simulink model "AutonomousTemplate_2020a"  (R2020a)
settings: Solver=ode23t  StartTime=0.0  StopTime=180.1  FixedStep=0.05  RelTol=1e-3  EnableMultiTasking=on
model workspace (MAT data in the model file):
  mapForSim : object (value not decoded)
  occGrid : robotics.BinaryOccupancyGrid (value not decoded)
undefined symbols (not defined in the file): cellLevel, cellPose, cellTypeArray, FloorSurface, isoPoses, platformPoses, PlowSurface, Ref, RobotSurface, WallSurface, X, Y, Z
libraries: sm_lib x286, nesl_utility x157, simulink x72, vexcommonlib x1
(part 15 of 15)

== stateflow chart AutonomousTemplate_2020a/Flow for robot movement ==
  note: At this point the Robot has done the entire left side for the field (looking out for where the robot start at) and needs to get to the left side. This is what this does
  note: This move the robot to the first box of cells and quickly moves into the movement program.
  state dispose3
    lach=0;
  state START
    Rmotor=0;
    Lmotor=0;
    scolev=1;
    i=0;
    tim=0;
    kim=0;
    c=0;
    cellin=0;
    lach=0;
    vac = 0;
    VCheck = 0;
  state Forward
    Rmotor=100;
    Lmotor=100;
  state Stop
    Rmotor = 0;
    Lmotor=0;
    scolev=0;
  state dispose1
    lach=0;
  note: After the robot does the sweep program before this it becomes a little off-center and need to return to the middle and that is done here.
  state dispose
    lach=0;
  state check7
    Rmotor=-50;
    Lmotor=50;
  state quit3
    Rmotor=0;
    Lmotor=0;
  state check3
    Rmotor=-50;
    Lmotor=50;
  state quit1
    Rmotor=0;
    Lmotor=0;
  note: After the robot does the sweep program before this it becomes a little off-center and need to return to the middle and that is done here.
  state Stop9
    Rmotor = 0;
    Lmotor=0;
  note: Second box isolating
  state Turn190
    Rmotor=27;
    Lmotor=-27;
  state Turn189
    Rmotor=29;
    Lmotor=-29;
  state Stop74
    Rmotor=0;
    Lmotor=0;
    lach=0;
  state Turn188
    Rmotor=29;
    Lmotor=-29;
  state correct
    Lmotor=25;
    Rmotor=0;
  state check1
    Rmotor=-50;
    Lmotor=50;
  state quit
    Rmotor=0;
    Lmotor=0;
  state dispose2
    lach=0;
  note: After the robot does the sweep program before this it becomes a little off-center and need to return to the middle and that is done here.
  state wat3
    Rmotor=0;
    Lmotor=0
  state Turn185
    Rmotor=27;
    Lmotor=-27;
  state Turn184
    Rmotor=29;
    Lmotor=-29;
  state Stop70
    Rmotor=0;
    Lmotor=0;
    lach=0;
  state Turn186
    Rmotor=29;
    Lmotor=-29;
  state Forward1
    Rmotor=50
    Lmotor=50;
    scolev=1;
  state Stop4
    Rmotor = 0;
    Lmotor=0;
  state Backwards
    Rmotor=-30;
    Lmotor=-30;
    scolev=0;
  state Stop6
    Rmotor = 0;
    Lmotor=0;
  state wat1
    Rmotor=0;
    Lmotor=0
  state Stop73
    Rmotor=50;
    Lmotor=50;
  state Turn191
    Rmotor=29;
    Lmotor=-29;
  state wat
    Rmotor=0;
    Lmotor=0
  state check5
    Rmotor=-50;
    Lmotor=50;
  state quit2
    Rmotor=0;
    Lmotor=0;
  state correct5
    Lmotor=25;
    Rmotor=0;
  state return1
    Lmotor=20;
    Rmotor=0;
  state Stop14
    Rmotor = 0;
    Lmotor=0;
  state check6
    Rmotor=50;
    Lmotor=-50;
  state Stop69
    Rmotor=0;
    Lmotor=0;
  state Turn187
    Rmotor=29;
    Lmotor=-29;
  state check2
    Rmotor=50;
    Lmotor=-50;
  state correct2
    Lmotor=25;
    Rmotor=0;
  state return
    Lmotor=20;
    Rmotor=0;
  state Stop12
    Rmotor = 0;
    Lmotor=0;
  note: It may seem that this 1 sec is not neceisary, but If I were to instantly transfer into the next state it would mess up my perfect 90-degree angle.
  note: after(1.4,sec)
  state check
    Rmotor=50;
    Lmotor=-50;
  state wat2
    Rmotor=0;
    Lmotor=0
  state drop
    Rmotor=50
    Lmotor=50;
    lach=0;
  state Turn90
    Rmotor=28.5;
    Lmotor=-28.5;
  state Stop5
    Rmotor = 0;
    Lmotor=0;
  state Vaccine
    vac = 1;
    Rmotor = 50;
    Lmotor = 50;
  state correct1
    Lmotor=0;
    Rmotor=25;
  state Backwards1
    Rmotor=-30;
    Lmotor=-30;
    scolev=0;
  state Vaccine3
    vac = 1;
    Rmotor = 50;
    Lmotor = 50;
  state Stop72
    Rmotor=50;
    Lmotor=50;
  state Vaccine1
    vac = 1;
    Rmotor = 50;
    Lmotor = 50;
  state check4
    Rmotor=50;
    Lmotor=-50;
  state Stop71
    Rmotor=0;
    Lmotor=0;
  state correct4
    Lmotor=0;
    Rmotor=25;
  state Backwards3
    Rmotor=-30;
    Lmotor=-30;
    scolev=0;
  state Vaccinate3
    Rmotor = -50;
    Lmotor = -50;
  state Vaccinate
    Rmotor = -50;
    Lmotor = -50;
  state Vaccinate1
    Rmotor = -50;
    Lmotor = -50;
  state correct3
    Lmotor=0;
    Rmotor=25;
  state Backwards2
    Rmotor=-30;
    Lmotor=-30;
    scolev=0;
  state Vaccine2
    vac = 1;
    Rmotor = 50;
    Lmotor = 50;
  note: This marks the START of the sweep program . The times are almost to the exact. make sure when using this you have the robot start at the correct place. otherwise the sweep will not work (by not covoring all possible spaces the may contain cells)
  note: This marks the START of the sweep program . The times are almost to the exact. make sure when using this you have the robot start at the correct place. otherwise the sweep will not work (by not covoring all possible spaces the may contain cells)
  note: This marks the START of the sweep program . The times are almost to the exact. make sure when using this you have the robot start at the correct place. otherwise the sweep will not work (by not covoring all possible spaces the may contain cells)
  note: This marks the START of the sweep program . The times are almost to the exact. make sure when using this you have the robot start at the correct place. otherwise the sweep will not work (by not covoring all possible spaces the may contain cells)
  note: when I refer to the sweep the dircetion movement refered to by L or R does NOT reflect the direction in which the robot rotates one motor?
  state Vaccinate2
    Rmotor = -50;
    Lmotor = -50;
  note: This marks the END of the sweep program ; when reused change the varibles so that it does not conflict.
  state Stop3
    Rmotor = 0;
    Lmotor=0;
    c=0;
    cellin=0;
    VCheck = 0;
  note: This marks the END of the sweep program ; when reused change the varibles so that it does not conflict.
  state Stop56
    Rmotor = 0;
    Lmotor=0;
    c=0;
    cellin=0;
  state Stop60
    Rmotor = 0;
    Lmotor=0;
    c=0;
    cellin=0;
  note: Troble Shoot
  note: This marks the END of the sweep program ; when reused change the varibles so that it does not conflict.
  state latch105
    i=1;
    lach=1;
    kim=time;
    cellin=1;
  state latch112
    i=1;
    lach=1;
    kim=time;
    cellin=1;
  state latch119
    i=1;
    lach=1;
    kim=time;
    cellin=1;
  state SweepR
    Rmotor=25;
    Lmotor=0;
  state time
    tim=time;
    c = c + 1;
    i=0;
  state SweepR84
    Rmotor=25;
    Lmotor=0;
  state time105
    tim=time;
    c = c + 1;
    i=0;
  state SweepR88
    Rmotor=25;
    Lmotor=0;
  state time112
    tim=time;
    c = c + 1;
    i=0;
  state SweepR92
    Rmotor=25;
    Lmotor=0;
  state time119
    tim=time;
    c = c + 1;
    i=0;
  state latch3
    i=1;
    lach=1;
    kim=time;
    cellin=1;
  state Stop58
    Rmotor = 0;
    Lmotor=0;
    c=0;
    cellin=0;
  state Reset
    Rmotor=50;
    Lmotor=50
    i=0;
  note: This marks the END of the sweep program ; when reused change the varibles so that it does not conflict.
  note: this is speific to this flow only and cannot be used on other sweeps
  state Stop57
    Rmotor = 0;
    Lmotor=0;
  state SweepL
    Rmotor=-22.5;
    Lmotor=25;
  state time1
    tim=time;
    c =c+1;
    i=0;
  state SweepL65
    Rmotor=-22.5;
    Lmotor=25;
  state time111
    tim=time;
    c =c+1;
    i=0;
  state SweepL68
    Rmotor=-22.5;
    Lmotor=25;
  state time118
    tim=time;
    c =c+1;
    i=0;
  state SweepL71
    Rmotor=-22.5;
    Lmotor=25;
  state time125
    tim=time;
    c =c+1;
    i=0;
  state latch106
    i=1;
    lach=1;
    kim=time;
    cellin==1;
  state latch113
    i=1;
    lach=1;
    kim=time;
    cellin==1;
  state latch120
    i=1;
    lach=1;
    kim=time;
    cellin==1;
  state latch
    i=1;
    lach=1;
    kim=time;
    cellin==1;
  state Stop1
    Rmotor = 0;
    Lmotor=0;
  state Stop59
    Rmotor = 0;
    Lmotor=0;
  state Stop61
    Rmotor = 0;
    Lmotor=0;
  note: after(.632,sec)
  state SweepR1
    Rmotor=25;
    Lmotor=-10;
  state time2
    tim=time;
    c = c + 1;
    i=0;
  state SweepR87
    Rmotor=25;
    Lmotor=-10;
  state time107
    tim=time;
    c = c + 1;
    i=0;
  state SweepR91
    Rmotor=25;
    Lmotor=-10;
  state time114
    tim=time;
    c = c + 1;
    i=0;
  state SweepR95
    Rmotor=25;
    Lmotor=-10;
  state time121
    tim=time;
    c = c + 1;
    i=0;
  state latch110
    i=1;
    lach=1;
    kim=time;
    cellin=1;
  state latch117
    i=1;
    lach=1;
    kim=time;
    cellin=1;
  state latch124
    i=1;
    lach=1;
    kim=time;
    cellin=1;
  state latch1
    i=1;
    lach=1;
    kim=time;
    cellin=1;
  state latch107
    i=1;
    lach=1;
    kim=time;
    cellin=1;
  state latch114
    i=1;
    lach=1;
    kim=time;
    cellin=1;
  state latch121
    i=1;
    lach=1;
    kim=time;
    cellin=1;
  state latch6
    i=1;
    lach=1;
    kim=time;
    cellin=1;
  state time4
    tim=time;
    c = c + 1;
    i=0;
  state time6
    tim=time;
    c = c + 1;
    i=0;
  state SweepR3
    Rmotor=25;
    Lmotor=-22.5;
  state time108
    tim=time;
    c = c + 1;
    i=0;
  state time109
    tim=time;
    c = c + 1;
    i=0;
  state SweepR86
    Rmotor=25;
    Lmotor=-22.5;
  state time115
    tim=time;
    c = c + 1;
    i=0;
  state time116
    tim=time;
    c = c + 1;
    i=0;
  state SweepR90
    Rmotor=25;
    Lmotor=-22.5;
  state time122
    tim=time;
    c = c + 1;
    i=0;
  state time123
    tim=time;
    c = c + 1;
    i=0;
  state SweepR94
    Rmotor=25;
    Lmotor=-22.5;
  state latch5
    i=1;
    lach=1;
    kim=time;
    cellin=1;
  state latch108
    i=1;
    lach=1;
    kim=time;
    cellin=1;
  state latch115
    i=1;
    lach=1;
    kim=time;
    cellin=1;
  state latch122
    i=1;
    lach=1;
    kim=time;
    cellin=1;
  state SweepL1
    Rmotor=-22.5;
    Lmotor=25;
  state SweepR2
    Rmotor=25;
    Lmotor=-10;
  state SweepL2
    Rmotor=-22.5;
    Lmotor=25;
  state latch109
    i=1;
    lach=1;
    kim=time;
    cellin=1;
  state SweepL63
    Rmotor=-22.5;
    Lmotor=25;
  state SweepR85
    Rmotor=25;
    Lmotor=-10;
  state SweepL64
    Rmotor=-22.5;
    Lmotor=25;
  state latch116
    i=1;
    lach=1;
    kim=time;
    cellin=1;
  state SweepL66
    Rmotor=-22.5;
    Lmotor=25;
  state SweepR89
    Rmotor=25;
    Lmotor=-10;
  state SweepL67
    Rmotor=-22.5;
    Lmotor=25;
  state latch123
    i=1;
    lach=1;
    kim=time;
    cellin=1;
  state SweepL69
    Rmotor=-22.5;
    Lmotor=25;
  state SweepR93
    Rmotor=25;
    Lmotor=-10;
  state SweepL70
    Rmotor=-22.5;
    Lmotor=25;
  state latch2
    i=1;
    lach=1;
    kim=time;
    cellin=1;
  state time3
    tim=time;
    c = c + 1;
    i=0;
  state time5
    tim=time;
    c = c + 1;
    i=0;
  state time106
    tim=time;
    c = c + 1;
    i=0;
  state latch111
    i=1;
    lach=1;
    kim=time;
    cellin=1;
  state time110
    tim=time;
    c = c + 1;
    i=0;
  state time113
    tim=time;
    c = c + 1;
    i=0;
  state latch118
    i=1;
    lach=1;
    kim=time;
    cellin=1;
  state time117
    tim=time;
    c = c + 1;
    i=0;
  state time120
    tim=time;
    c = c + 1;
    i=0;
  state latch125
    i=1;
    lach=1;
    kim=time;
    cellin=1;
  state time124
    tim=time;
    c = c + 1;
    i=0;
  state latch4
    i=1;
    lach=1;
    kim=time;
    cellin=1;
  state Drop2
    lach = 0;
  state check10
    Rmotor=-50;
    Lmotor=50;
  note: The values are slightly diffrent to account for uncentering during the 180 degree rotation
  note: 3.6 second for next grid line on the specific transition
  state check12
    Rmotor=-50;
    Lmotor=50;
  state check8
    Rmotor=-50;
    Lmotor=50;
  state Rotate2
    Rmotor = 50;
    Lmotor = -50;
  state dispose5
    lach=0;
  state dispose6
    lach=0;
  state Backwards5
    Rmotor=-30;
    Lmotor=-30;
    scolev=0;
  state correct9
    Lmotor=0;
    Rmotor=25;
  state wat5
    Rmotor=0;
    Lmotor=0
  state Forward5
    Rmotor = 50;
    Lmotor = 50;
  state Drop
    lach = 0;
  state Stop17
    Rmotor=0;
    Lmotor=0;
  state Forward2
    Rmotor=50;
    Lmotor=50.7;
  state Turn181
    Rmotor=27;
    Lmotor=-27;
  note: At this point the Robot has done the entire left side for the field (looking out for where the robot start at) and needs to get to the left side. This is what this does
  state Stop24
    Rmotor = 0;
    Lmotor=0;
  state Turn183
    Rmotor=27;
    Lmotor=-27;
  state dispose4
    lach=0;
  state quit5
    Rmotor=0;
    Lmotor=0;
  state wat6
    Rmotor=0;
    Lmotor=0
  state check11
    Rmotor=50;
    Lmotor=-50;
  state Backwards4
    Rmotor=-30;
    Lmotor=-30;
    scolev=0;
  state correct7
    Lmotor=0;
    Rmotor=25;
  state quit6
    Rmotor=0;
    Lmotor=0;
  state wat4
    Rmotor=0;
    Lmotor=0
  state check13
    Rmotor=50;
    Lmotor=-50;
  state Rotate3
    Rmotor = -50;
    Lmotor = 50;
  state Vaccine5
    vac = 1;
    Rmotor = 50;
    Lmotor = 50;
  state quit4
    Rmotor=0;
    Lmotor=0;
  state check9
    Rmotor=50;
    Lmotor=-50;
  state Vaccine6
    vac = 1;
    Rmotor = 50;
    Lmotor = 50;
  note: Had to re-arrange this program to from right to left. refer to here if you need antoher format like this, otherwise use the others.
  state Drop1
    lach = 0;
  state Rotate
    Rmotor = -50;
    Lmotor = 50;
  state Stop16
    Rmotor=0;
    Lmotor=0;
  state Turn182
    Rmotor=29;
    Lmotor=-29;
  state Backwards7
    Rmotor=-30;
    Lmotor=-30;
    scolev=0;
  state correct11
    Lmotor=0;
    Rmotor=25;
  state Rotate1
    Rmotor = 50;
    Lmotor = -50;
  state Vaccinate5
    Rmotor = -50;
    Lmotor = -50;
  state Vaccine4
    vac = 1;
    Rmotor = 50;
    Lmotor = 50;
  state Stop25
    Rmotor = 0;
    Lmotor=0;
  state Backwards6
    Rmotor=-30;
    Lmotor=-30;
    scolev=0;
  state Stop23
    Rmotor = 0;
    Lmotor=0;
  state Forward4
    Lmotor=50;
    Rmotor=50;
  state Stop22
    Rmotor = 0;
    Lmotor=0;
  state correct8
    Lmotor=25;
    Rmotor=0;
  state Vaccinate6
    Rmotor = -50;
    Lmotor = -50;
  state Stop20
    Rmotor = 0;
    Lmotor=0;
  state correct6
    Lmotor=25;
    Rmotor=0;
  note: This marks the START of the sweep program . The times are almost to the exact. make sure when using this you have the robot start at the correct place. otherwise the sweep will not work (by not covoring all possible spaces the may contain cells)
  state Vaccinate4
    Rmotor = -50;
    Lmotor = -50;
  state DropStart
    Rmotor = 50;
    Lmotor = -50;
  state Stop27
    Rmotor = 0;
    Lmotor=0;
  state correct10
    Lmotor=25;
    Rmotor=0;
  state Stop64
    Rmotor = 0;
    Lmotor=0;
    c=0;
    cellin=0;
  note: This marks the END of the sweep program ; when reused change the varibles so that it does not conflict.
  note: This marks the START of the sweep program . The times are almost to the exact. make sure when using this you have the robot start at the correct place. otherwise the sweep will not work (by not covoring all possible spaces the may contain cells)
  state latch133
    i=1;
    lach=1;
    kim=time;
    cellin=1;
  state SweepR103
    Rmotor=25;
    Lmotor=0;
  state time134
    tim=time;
    c = c + 1;
    i=0;
  state Stop62
    Rmotor = 0;
    Lmotor=0;
    c=0;
    cellin=0;
  note: This marks the END of the sweep program ; when reused change the varibles so that it does not conflict.
  note: This marks the START of the sweep program . The times are almost to the exact. make sure when using this you have the robot start at the correct place. otherwise the sweep will not work (by not covoring all possible spaces the may contain cells)
  state Forward6
    Rmotor = 50;
    Lmotor = 50;
  state latch126
    i=1;
    lach=1;
    kim=time;
    cellin=1;
  state SweepR96
    Rmotor=25;
    Lmotor=0;
  state time126
    tim=time;
    c = c + 1;
    i=0;
  state Stop66
    Rmotor = 0;
    Lmotor=0;
    c=0;
    cellin=0;
  note: This marks the END of the sweep program ; when reused change the varibles so that it does not conflict.
  state latch140
    i=1;
    lach=1;
    kim=time;
    cellin=1;
  state SweepR107
    Rmotor=25;
    Lmotor=0;
  state time141
    tim=time;
    c = c + 1;
    i=0;
  state SweepL75
    Rmotor=-22.5;
    Lmotor=25;
  state time133
    tim=time;
    c =c+1;
    i=0;
  state latch139
    i=1;
    lach=1;
    kim=time;
    cellin==1;
  state Drop3
    Rmotor = 0;
    Lmotor = 0;
    lach = 0;
  state Stop65
    Rmotor = 0;
    Lmotor=0;
  state Turn
    Rmotor = 50;
    Lmotor = -50;
  state SweepL74
    Rmotor=-22.5;
    Lmotor=25;
  state time132
    tim=time;
    c =c+1;
    i=0;
  state latch127
    i=1;
    lach=1;
    kim=time;
    cellin==1;
  state Stop63
    Rmotor = 0;
    Lmotor=0;
  state latch138
    i=1;
    lach=1;
    kim=time;
    cellin=1;
  state SweepR102
    Rmotor=25;
    Lmotor=-10;
  state time137
    tim=time;
    c = c + 1;
    i=0;
  state SweepL78
    Rmotor=-22.5;
    Lmotor=25;
  state time140
    tim=time;
    c =c+1;
    i=0;
  state latch135
    i=1;
    lach=1;
    kim=time;
    cellin=1;
  state latch146
    i=1;
    lach=1;
    kim=time;
    cellin==1;
  state SweepR101
    Rmotor=25;
    Lmotor=-22.5;
  state time138
    tim=time;
    c = c + 1;
    i=0;
  state time139
    tim=time;
    c = c + 1;
    i=0;
  state Stop67
    Rmotor = 0;
    Lmotor=0;
  state latch131
    i=1;
    lach=1;
    kim=time;
    cellin=1;
  state SweepR99
    Rmotor=25;
    Lmotor=-10;
  state time128
    tim=time;
    c = c + 1;
    i=0;
  state latch128
    i=1;
    lach=1;
    kim=time;
    cellin=1;
  state SweepR98
    Rmotor=25;
    Lmotor=-22.5;
  state time129
    tim=time;
    c = c + 1;
    i=0;
  state time130
    tim=time;
    c = c + 1;
    i=0;
  state latch134
    i=1;
    lach=1;
    kim=time;
    cellin=1;
  state latch137
    i=1;
    lach=1;
    kim=time;
    cellin=1;
  state SweepL76
    Rmotor=-22.5;
    Lmotor=25;
  state SweepR100
    Rmotor=25;
    Lmotor=-10;
  state SweepL77
    Rmotor=-22.5;
    Lmotor=25;
  state latch145
    i=1;
    lach=1;
    kim=time;
    cellin=1;
  state SweepR106
    Rmotor=25;
    Lmotor=-10;
  state time144
    tim=time;
    c = c + 1;
    i=0;
  state latch142
    i=1;
    lach=1;
    kim=time;
    cellin=1;
  state SweepR105
    Rmotor=25;
    Lmotor=-22.5;
  state time145
    tim=time;
    c = c + 1;
    i=0;
  state time146
    tim=time;
    c = c + 1;
    i=0;
  state latch130
    i=1;
    lach=1;
    kim=time;
    cellin=1;
  state latch129
    i=1;
    lach=1;
    kim=time;
    cellin=1;
  state SweepL73
    Rmotor=-22.5;
    Lmotor=25;
  state SweepR97
    Rmotor=25;
    Lmotor=-10;
  state SweepL72
    Rmotor=-22.5;
    Lmotor=25;
  state latch141
    i=1;
    lach=1;
    kim=time;
    cellin=1;
  state latch144
    i=1;
    lach=1;
    kim=time;
    cellin=1;
  state time136
    tim=time;
    c = c + 1;
    i=0;
  state latch136
    i=1;
    lach=1;
    kim=time;
    cellin=1;
  state time135
    tim=time;
    c = c + 1;
    i=0;
  state SweepL79
    Rmotor=-22.5;
    Lmotor=25;
  state SweepR104
    Rmotor=25;
    Lmotor=-10;
  state SweepL80
    Rmotor=-22.5;
    Lmotor=25;
  state time131
    tim=time;
    c = c + 1;
    i=0;
  state latch132
    i=1;
    lach=1;
    kim=time;
    cellin=1;
  state time127
    tim=time;
    c = c + 1;
    i=0;
  state time143
    tim=time;
    c = c + 1;
    i=0;
  state latch143
    i=1;
    lach=1;
    kim=time;
    cellin=1;
  state time142
    tim=time;
    c = c + 1;
    i=0;
  (default) -> START
  dispose3 -> check7
  dispose1 -> check3
  START -> Forward
  Forward -> Stop : after(2.68,sec)
  quit3 -> correct5 : after(.2,sec)
  wat3 -> dispose3 [order 1] : after(1,sec)[ctype~=2]
  dispose -> check1
  Stop -> SweepR
  wat1 -> dispose1 [order 1] : after(1,sec)[ctype~=2]
  quit1 -> correct : after(.2,sec)
  check7 -> quit3 : after(1,sec)
  wat -> dispose [order 1] : after(1,sec)[ctype==1 || ctype==0]
  check3 -> quit1 : after(1,sec)
  Stop9 -> Turn185 [order 2] : [lach==1]
  quit -> Forward1 : after(.2,sec)
  wat3 -> check7 [order 2] : after(1,sec)[ctype==2]
  dispose2 -> check5
  Stop9 -> SweepR88 [order 1] : [lach==0]
  Stop12 -> Turn190 [order 2] : [lach == 1]
  Stop74 -> Turn188 : after(.2,sec)
  Turn190 -> Turn189 : after(3,sec)
  check1 -> quit : after(1,sec)
  wat1 -> check3 [order 2] : after(1,sec)[ctype==2]
  Stop56 -> correct [order 1] : [lach==0]
  quit2 -> correct2 : after(.2,sec)
  Backwards1 -> Stop9 : after(0.4,sec)
  Turn189 -> Stop73 : [ang<105]
  Stop73 -> Stop74 : after(1.5,sec)
  Turn188 -> Turn191 : after(3,sec)
  Stop70 -> Turn186 : after(.2,sec)
  Turn185 -> Turn184 : after(3,sec)
  correct -> correct1 : after(1,sec)
  wat -> check1 [order 2] : after(1,sec)[ctype==2]
  wat2 -> dispose2 [order 1] : after(1,sec)[ctype~=2]
  drop -> Stop4 : after(.7,sec)
  Backwards -> Stop6 : after(0.85,sec)
  Stop6 -> SweepR84
  Stop3 -> Forward1 [order 1] : [lach==0]
  check6 -> wat3 : after(1,sec)
  Turn184 -> Stop69 : [ang<105]
  Stop69 -> Stop70 : after(.2,sec)
  Turn186 -> Turn187 : after(3,sec)
  check5 -> quit2 : after(1,sec)
  Forward1 -> drop : after(.7,sec)
  Stop4 -> Turn90
  Stop5 -> Backwards : after(0.3,sec)
  Stop60 -> correct5 [order 1] : [lach == 0]
  return1 -> Stop14 : after(.001,sec)
  check2 -> wat1 : after(1,sec)
  Stop14 -> Turn181
  Turn191 -> Stop72 : [ang>75]
  check -> wat : after(1,sec)
  Stop58 -> correct2 [order 1] : [lach == 0]
  wat2 -> check5 [order 2] : after(1,sec)[ctype==2]
  return -> Stop12 : after(.2,sec)
  correct5 -> correct4 : after(1,sec)
  Backwards3 -> return1 : after(.45,sec)
  Stop12 -> SweepR92 [order 1] : [lach == 0]
  Vaccine3 -> check6 : after(1, sec){vac = 0;}
  Turn187 -> Stop71 : [ang>75]
  Vaccine1 -> check2 : after(1, sec){vac = 0;}
  correct2 -> correct3 : after(1,sec)
  Backwards2 -> return : after(.45,sec)
  Vaccine -> check : after(1, sec){vac = 0;}
  Turn90 -> Stop5 : [ang>75]
  check4 -> wat2 : after(1,sec)
  correct1 -> Backwards1 : after(1,sec)
  Stop72 -> SweepR92 : after(1.5, sec)
  Vaccinate -> Vaccine : after(1, sec)
  Vaccinate3 -> Vaccine3 : after(1, sec)
  Stop71 -> SweepR88
  Vaccinate1 -> Vaccine1 : after(1, sec)
  Vaccine2 -> check4 : after(1, sec){vac = 0;}
  correct4 -> Backwards3 : after(1,sec)
  Stop60 -> Vaccinate3 [order 2] : [lach==1]
  correct3 -> Backwards2 : after(1,sec)
  Stop56 -> Vaccinate1 [order 2] : [lach==1]
  Stop3 -> Vaccinate [order 2] : [lach==1]
  Vaccinate2 -> Vaccine2 : after(1, sec)
  Stop58 -> Vaccinate2 [order 2] : [lach==1]
  SweepR84 -> latch105 [order 2] : [cellin==0 && i==0 && ctype==2]
  SweepR88 -> latch112 [order 2] : [cellin==0 && i==0 && ctype==2]
  SweepR92 -> latch119 [order 2] : [cellin==0 && i==0 && ctype==2]
  Stop61 -> Stop60
  SweepR -> time [order 1] : [c==0]
  SweepR84 -> time105 [order 1] : [c==0]
  SweepR88 -> time112 [order 1] : [c==0]
  SweepR92 -> time119 [order 1] : [c==0]
  Stop57 -> Stop56 : after(.2,sec)
  SweepR -> latch3 [order 2] : [cellin==0 && i==0 && ctype==2]
  Reset -> Stop3 : after(.667,sec)
  latch105 -> SweepR84
  latch112 -> SweepR88
  latch119 -> SweepR92
  latch3 -> SweepR
  time -> SweepR
  time105 -> SweepR84
  time112 -> SweepR88
  time119 -> SweepR92
  SweepR -> SweepL [order 4] : after(1.24-(kim-tim),sec)[i==1]
  SweepR -> SweepL [order 3] : after(1.24,sec)[i==0]
  SweepR84 -> SweepL65 [order 4] : after(1.24-(kim-tim),sec)[i==1]
  SweepR84 -> SweepL65 [order 3] : after(1.24,sec)[i==0]
  SweepR88 -> SweepL68 [order 4] : after(1.24-(kim-tim),sec)[i==1]
  SweepR88 -> SweepL68 [order 3] : after(1.24,sec)[i==0]
  SweepR92 -> SweepL71 [order 4] : after(1.24-(kim-tim),sec)[i==1]
  SweepR92 -> SweepL71 [order 3] : after(1.24,sec)[i==0]
  Stop59 -> Stop58
  Stop1 -> Reset
  SweepL65 -> latch106 [order 2] : [cellin==0 && i==0 && ctype==2]
  SweepL68 -> latch113 [order 2] : [cellin==0 && i==0 && ctype==2]
  SweepL71 -> latch120 [order 2] : [cellin==0 && i==0 && ctype==2]
  SweepL -> time1 [order 1] : [c==1]
  SweepL65 -> time111 [order 1] : [c==1]
  SweepL68 -> time118 [order 1] : [c==1]
  SweepL71 -> time125 [order 1] : [c==1]
  SweepL -> latch [order 2] : [cellin==0 && i==0 && ctype==2]
  SweepR86 -> Stop57 [order 3] : after(.7,sec)[i==0]
  SweepR86 -> Stop57 [order 4] : after(.7-(kim-tim),sec)[i==1]
  time1 -> SweepL
  time111 -> SweepL65
  time118 -> SweepL68
  time125 -> SweepL71
  latch -> SweepL
  latch106 -> SweepL65
  latch113 -> SweepL68
  latch120 -> SweepL71
  SweepL -> SweepR1 [order 4] : after(1.55-(kim-tim),sec)[i==1]
  SweepL -> SweepR1 [order 3] : after(1.55,sec)[i==0]
  SweepL65 -> SweepR87 [order 4] : after(1.55-(kim-tim),sec)[i==1]
  SweepL65 -> SweepR87 [order 3] : after(1.55,sec)[i==0]
  SweepL68 -> SweepR91 [order 4] : after(1.55-(kim-tim),sec)[i==1]
  SweepL68 -> SweepR91 [order 3] : after(1.55,sec)[i==0]
  SweepL71 -> SweepR95 [order 4] : after(1.55-(kim-tim),sec)[i==1]
  SweepL71 -> SweepR95 [order 3] : after(1.55,sec)[i==0]
  SweepR3 -> Stop1 [order 3] : after(.7,sec)[i==0]
  SweepR3 -> Stop1 [order 4] : after(.7-(kim-tim),sec)[i==1]
  SweepR90 -> Stop59 [order 3] : after(.7,sec)[i==0]
  SweepR90 -> Stop59 [order 4] : after(.7-(kim-tim),sec)[i==1]
  SweepR94 -> Stop61 [order 3] : after(.7,sec)[i==0]
  SweepR94 -> Stop61 [order 4] : after(.7-(kim-tim),sec)[i==1]
  SweepR1 -> time2 [order 1] : [c==2]
  SweepR87 -> time107 [order 1] : [c==2]
  SweepR91 -> time114 [order 1] : [c==2]
  SweepR95 -> time121 [order 1] : [c==2]
  SweepR1 -> latch1 [order 2] : [cellin==0 && i==0 && ctype==2]
  SweepR87 -> latch107 [order 2] : [cellin==0 && i==0 && ctype==2]
  SweepR91 -> latch114 [order 2] : [cellin==0 && i==0 && ctype==2]
  SweepR95 -> latch121 [order 2] : [cellin==0 && i==0 && ctype==2]
  latch110 -> SweepR86
  latch117 -> SweepR90
  latch124 -> SweepR94
  time6 -> SweepR3
  time109 -> SweepR86
  time116 -> SweepR90
  time123 -> SweepR94
  latch6 -> SweepR3
  time2 -> SweepR1
  time107 -> SweepR87
  time114 -> SweepR91
  time121 -> SweepR95
  latch1 -> SweepR1
  SweepR86 -> latch110 [order 2] : [cellin==0 && i==0 && ctype==2]
  SweepR90 -> latch117 [order 2] : [cellin==0 && i==0 && ctype==2]
  SweepR94 -> latch124 [order 2] : [cellin==0 && i==0 && ctype==2]
  latch107 -> SweepR87
  latch114 -> SweepR91
  latch121 -> SweepR95
  SweepR3 -> latch6 [order 2] : [cellin==0 && i==0 && ctype==2]
  SweepR3 -> time6 [order 1] : [c==5]
  SweepR86 -> time109 [order 1] : [c==5]
  SweepR90 -> time116 [order 1] : [c==5]
  SweepR94 -> time123 [order 1] : [c==5]
  SweepR1 -> SweepL1 [order 4] : after(2.348-(kim-tim),sec)[i==1]
  SweepR1 -> SweepL1 [order 3] : after(2.348,sec)[i==0]
  SweepR87 -> SweepL63 [order 4] : after(2.348-(kim-tim),sec)[i==1]
  SweepR87 -> SweepL63 [order 3] : after(2.348,sec)[i==0]
  SweepR91 -> SweepL66 [order 4] : after(2.348-(kim-tim),sec)[i==1]
  SweepR91 -> SweepL66 [order 3] : after(2.348,sec)[i==0]
  SweepR95 -> SweepL69 [order 4] : after(2.348-(kim-tim),sec)[i==1]
  SweepR95 -> SweepL69 [order 3] : after(2.348,sec)[i==0]
  SweepR2 -> time4 [order 1] : [c==4]
  time4 -> SweepR2
  SweepL2 -> SweepR3 [order 3] : after(1.5,sec)[i==0]
  SweepL2 -> SweepR3 [order 4] : after(1.5-(kim-tim),sec)[i==1]
  SweepR85 -> time108 [order 1] : [c==4]
  time108 -> SweepR85
  SweepL64 -> SweepR86 [order 3] : after(1.5,sec)[i==0]
  SweepL64 -> SweepR86 [order 4] : after(1.5-(kim-tim),sec)[i==1]
  SweepR89 -> time115 [order 1] : [c==4]
  time115 -> SweepR89
  SweepL67 -> SweepR90 [order 3] : after(1.5,sec)[i==0]
  SweepL67 -> SweepR90 [order 4] : after(1.5-(kim-tim),sec)[i==1]
  SweepR93 -> time122 [order 1] : [c==4]
  time122 -> SweepR93
  SweepL70 -> SweepR94 [order 3] : after(1.5,sec)[i==0]
  SweepL70 -> SweepR94 [order 4] : after(1.5-(kim-tim),sec)[i==1]
  SweepL63 -> latch109 [order 2] : [cellin==0 && i==0 && ctype==2]
  SweepL66 -> latch116 [order 2] : [cellin==0 && i==0 && ctype==2]
  SweepL69 -> latch123 [order 2] : [cellin==0 && i==0 && ctype==2]
  latch108 -> SweepL64
  latch115 -> SweepL67
  latch122 -> SweepL70
  latch5 -> SweepL2
  SweepL1 -> latch2 [order 2] : [cellin==0 && i==0 && ctype==2]
  SweepL1 -> SweepR2 [order 3] : after(1.42,sec)[i==0]
  SweepL63 -> SweepR85 [order 3] : after(1.42,sec)[i==0]
  SweepL66 -> SweepR89 [order 3] : after(1.42,sec)[i==0]
  SweepL69 -> SweepR93 [order 3] : after(1.42,sec)[i==0]
  SweepR2 -> SweepL2 [order 3] : after(1.923342,sec)[i==0]
  SweepR85 -> SweepL64 [order 3] : after(1.923342,sec)[i==0]
  SweepR89 -> SweepL67 [order 3] : after(1.923342,sec)[i==0]
  SweepR93 -> SweepL70 [order 3] : after(1.923342,sec)[i==0]
  SweepL1 -> SweepR2 [order 4] : after(1.42-(kim-tim),sec)[i==1]
  SweepL63 -> SweepR85 [order 4] : after(1.42-(kim-tim),sec)[i==1]
  SweepL66 -> SweepR89 [order 4] : after(1.42-(kim-tim),sec)[i==1]
  SweepL69 -> SweepR93 [order 4] : after(1.42-(kim-tim),sec)[i==1]
  SweepR2 -> SweepL2 [order 4] : after(1.923342-(kim-tim),sec)[i==1]
  SweepR85 -> SweepL64 [order 4] : after(1.923342-(kim-tim),sec)[i==1]
  SweepR89 -> SweepL67 [order 4] : after(1.923342-(kim-tim),sec)[i==1]
  SweepR93 -> SweepL70 [order 4] : after(1.923342-(kim-tim),sec)[i==1]
  latch109 -> SweepL63
  latch116 -> SweepL66
  latch123 -> SweepL69
  SweepL64 -> latch108 [order 2] : [cellin==0 && i==0 && ctype==2]
  SweepL67 -> latch115 [order 2] : [cellin==0 && i==0 && ctype==2]
  SweepL70 -> latch122 [order 2] : [cellin==0 && i==0 && ctype==2]
  SweepL2 -> latch5 [order 2] : [cellin==0 && i==0 && ctype==2]
  latch2 -> SweepL1
  SweepL1 -> time3 [order 1] : [c==3]
  time3 -> SweepL1
  SweepR2 -> latch4 [order 2] : [cellin==0 && i==0 && ctype==2]
  latch4 -> SweepR2
  time5 -> SweepL2
  SweepL2 -> time5 [order 1] : [c==5]
  SweepL63 -> time106 [order 1] : [c==3]
  time106 -> SweepL63
  SweepR85 -> latch111 [order 2] : [cellin==0 && i==0 && ctype==2]
  latch111 -> SweepR85
  time110 -> SweepL64
  SweepL64 -> time110 [order 1] : [c==5]
  SweepL66 -> time113 [order 1] : [c==3]
  time113 -> SweepL66
  SweepR89 -> latch118 [order 2] : [cellin==0 && i==0 && ctype==2]
  latch118 -> SweepR89
  time117 -> SweepL67
  SweepL67 -> time117 [order 1] : [c==5]
  SweepL69 -> time120 [order 1] : [c==3]
  time120 -> SweepL69
  SweepR93 -> latch125 [order 2] : [cellin==0 && i==0 && ctype==2]
  latch125 -> SweepR93
  time124 -> SweepL70
  SweepL70 -> time124 [order 1] : [c==5]
  wat5 -> check10 [order 2] : after(1,sec)[ctype==2]
  Drop2 -> Rotate2
  check10 -> quit5 : after(1,sec)
  Forward5 -> Drop2 : after(1, sec)
  wat6 -> check12 [order 2] : after(1,sec)[ctype==2]
  dispose5 -> check10
  check12 -> quit6 : after(1,sec)
  wat4 -> check8 [order 2] : after(1,sec)[ctype==2]
  dispose6 -> check12
  Rotate2 -> Forward4 : after(2.25, sec)
  check8 -> quit4 : after(1,sec)
  wat5 -> dispose5 [order 1] : after(1,sec)[ctype~=2]
  dispose4 -> check8
  wat6 -> dispose6 [order 1] : after(1,sec)[ctype~=2]
  check11 -> wat5 : after(1,sec)
  correct9 -> Backwards5 : after(1,sec)
  Forward2 -> Drop : after(2.5, sec)
  Drop -> Stop17 : after(0.59,sec)
  Stop17 -> SweepR96
  wat4 -> dispose4 [order 1] : after(1,sec)[ctype~=2]
  Turn183 -> Stop24 : [ang<15]
  Backwards5 -> Stop22 : after(0.4,sec)
  correct8 -> correct9 : after(1,sec)
  check13 -> wat6 : after(1,sec)
  Rotate3 -> Forward5 : after(2.25, sec)
  Stop16 -> Forward2 : after(.5,sec)
  Turn181 -> Turn182 : after(3,sec)
  Stop24 -> Backwards6 : after(.2,sec)
  Stop23 -> Turn183 : after(.2,sec)
  Vaccine5 -> check11 : after(1, sec){vac = 0;}
  quit5 -> correct8 : after(.2,sec)
  correct7 -> Backwards4 : after(1,sec)
  check9 -> wat4 : after(1,sec)
  Backwards4 -> Stop20 : after(0.4,sec)
  correct6 -> correct7 : after(1,sec)
  Vaccine6 -> check13 : after(1, sec){vac = 0;}
  Stop22 -> Rotate3 [order 2] : [lach == 1]
  quit6 -> correct10 : after(.2,sec)
  Vaccinate5 -> Vaccine5 : after(1, sec)
  Drop1 -> Rotate1
  Vaccine4 -> check9 : after(1, sec){vac = 0;}
  quit4 -> correct6 : after(.2,sec)
  Stop20 -> Rotate [order 2] : [lach == 1]
  Turn182 -> Stop16 : [ang<105]
  correct11 -> Backwards7 : after(1,sec)
  Rotate -> Drop1 : after(2.5, sec)
  Stop64 -> Vaccinate5 [order 2] : [lach==1]
  Rotate1 -> SweepR103 : after(2.5, sec)
  Vaccinate6 -> Vaccine6 : after(1, sec)
  Stop64 -> correct8 [order 1] : [lach == 0]
  Backwards6 -> Stop25 : after(0.61,sec)
  Forward4 -> Stop23 : after(2.85,sec)
  Backwards7 -> Stop27 : after(0.4,sec)
  correct10 -> correct11 : after(1,sec)
  Stop22 -> Forward4 [order 1] : after(.2,sec)
  Stop25 -> SweepR107
  Vaccinate4 -> Vaccine4 : after(1, sec)
  Stop66 -> Vaccinate6 [order 2] : [lach==1]
  Stop62 -> correct6 [order 1] : [lach == 0]
  Stop20 -> SweepR103 [order 1] : [lach == 0]
  Stop62 -> Vaccinate4 [order 2] : [lach==1]
  Stop66 -> correct10 [order 1] : [lach == 0]
  Stop27 -> DropStart
  DropStart -> Forward6 : after(1.125, sec)
  SweepR103 -> latch133 [order 2] : [cellin==0 && i==0 && ctype==2]
  SweepR103 -> time134 [order 1] : [c==0]
  Stop65 -> Stop64
  latch133 -> SweepR103
  time134 -> SweepR103
  SweepR103 -> SweepL75 [order 4] : after(1.24-(kim-tim),sec)[i==1]
  SweepR103 -> SweepL75 [order 3] : after(1.24,sec)[i==0]
  SweepR96 -> latch126 [order 2] : [cellin==0 && i==0 && ctype==2]
  SweepR96 -> time126 [order 1] : [c==0]
  Stop63 -> Stop62
  latch126 -> SweepR96
  time126 -> SweepR96
  Forward6 -> Turn : after(3, sec)
  SweepR96 -> SweepL74 [order 4] : after(1.24-(kim-tim),sec)[i==1]
  SweepR96 -> SweepL74 [order 3] : after(1.24,sec)[i==0]
  SweepR107 -> latch140 [order 2] : [cellin==0 && i==0 && ctype==2]
  SweepR107 -> time141 [order 1] : [c==0]
  Stop67 -> Stop66
  SweepL75 -> latch139 [order 2] : [cellin==0 && i==0 && ctype==2]
  SweepL75 -> time133 [order 1] : [c==1]
  latch140 -> SweepR107
  time141 -> SweepR107
  time133 -> SweepL75
  latch139 -> SweepL75
  Turn -> Drop3 : after(0.25,sec)
  SweepR107 -> SweepL78 [order 4] : after(1.24-(kim-tim),sec)[i==1]
  SweepR107 -> SweepL78 [order 3] : after(1.24,sec)[i==0]
  SweepL75 -> SweepR102 [order 4] : after(1.55-(kim-tim),sec)[i==1]
  SweepL75 -> SweepR102 [order 3] : after(1.55,sec)[i==0]
  SweepL74 -> latch127 [order 2] : [cellin==0 && i==0 && ctype==2]
  SweepL74 -> time132 [order 1] : [c==1]
  SweepR101 -> Stop65 [order 3] : after(.7,sec)[i==0]
  SweepR101 -> Stop65 [order 4] : after(.7-(kim-tim),sec)[i==1]
  time132 -> SweepL74
  latch127 -> SweepL74
  SweepL74 -> SweepR99 [order 4] : after(1.55-(kim-tim),sec)[i==1]
  SweepL74 -> SweepR99 [order 3] : after(1.55,sec)[i==0]
  SweepR102 -> time137 [order 1] : [c==2]
  SweepR102 -> latch135 [order 2] : [cellin==0 && i==0 && ctype==2]
  SweepR101 -> latch138 [order 2] : [cellin==0 && i==0 && ctype==2]
  SweepR98 -> Stop63 [order 3] : after(.7,sec)[i==0]
  SweepR98 -> Stop63 [order 4] : after(.7-(kim-tim),sec)[i==1]
  SweepL78 -> latch146 [order 2] : [cellin==0 && i==0 && ctype==2]
  SweepL78 -> time140 [order 1] : [c==1]
  SweepR101 -> time139 [order 1] : [c==5]
  time137 -> SweepR102
  latch138 -> SweepR101
  time140 -> SweepL78
  latch135 -> SweepR102
  time139 -> SweepR101
  latch146 -> SweepL78
  SweepR102 -> SweepL77 [order 4] : after(2.348-(kim-tim),sec)[i==1]
  SweepR102 -> SweepL77 [order 3] : after(2.348,sec)[i==0]
  SweepL78 -> SweepR106 [order 4] : after(1.55-(kim-tim),sec)[i==1]
  SweepL78 -> SweepR106 [order 3] : after(1.55,sec)[i==0]
  SweepL76 -> SweepR101 [order 3] : after(1.5,sec)[i==0]
  SweepL76 -> SweepR101 [order 4] : after(1.5-(kim-tim),sec)[i==1]
  SweepR100 -> time138 [order 1] : [c==4]
  time138 -> SweepR100
  SweepR99 -> time128 [order 1] : [c==2]
  SweepR99 -> latch128 [order 2] : [cellin==0 && i==0 && ctype==2]
  SweepR98 -> latch131 [order 2] : [cellin==0 && i==0 && ctype==2]
  SweepR98 -> time130 [order 1] : [c==5]
  time128 -> SweepR99
  SweepR105 -> Stop67 [order 3] : after(.7,sec)[i==0]
  SweepR105 -> Stop67 [order 4] : after(.7-(kim-tim),sec)[i==1]
  latch131 -> SweepR98
  latch128 -> SweepR99
  time130 -> SweepR98
  SweepR99 -> SweepL72 [order 4] : after(2.348-(kim-tim),sec)[i==1]
  SweepR99 -> SweepL72 [order 3] : after(2.348,sec)[i==0]
  SweepL73 -> SweepR98 [order 3] : after(1.5,sec)[i==0]
  SweepL73 -> SweepR98 [order 4] : after(1.5-(kim-tim),sec)[i==1]
  SweepR97 -> time129 [order 1] : [c==4]
  time129 -> SweepR97
  SweepR100 -> SweepL76 [order 4] : after(1.923342-(kim-tim),sec)[i==1]
  SweepL76 -> latch137 [order 2] : [cellin==0 && i==0 && ctype==2]
  latch134 -> SweepL77
  SweepL77 -> SweepR100 [order 4] : after(1.42-(kim-tim),sec)[i==1]
  SweepR106 -> time144 [order 1] : [c==2]
  SweepR106 -> latch142 [order 2] : [cellin==0 && i==0 && ctype==2]
  SweepR105 -> latch145 [order 2] : [cellin==0 && i==0 && ctype==2]
  SweepR105 -> time146 [order 1] : [c==5]
  SweepR100 -> SweepL76 [order 3] : after(1.923342,sec)[i==0]
  SweepL77 -> SweepR100 [order 3] : after(1.42,sec)[i==0]
  SweepL77 -> latch134 [order 2] : [cellin==0 && i==0 && ctype==2]
  latch137 -> SweepL76
  time144 -> SweepR106
  latch145 -> SweepR105
  latch142 -> SweepR106
  time136 -> SweepL76
  SweepL76 -> time136 [order 1] : [c==5]
  SweepR100 -> latch136 [order 2] : [cellin==0 && i==0 && ctype==2]
  latch136 -> SweepR100
  SweepL77 -> time135 [order 1] : [c==3]
  time135 -> SweepL77
  time146 -> SweepR105
  SweepR106 -> SweepL80 [order 4] : after(2.348-(kim-tim),sec)[i==1]
  SweepR106 -> SweepL80 [order 3] : after(2.348,sec)[i==0]
  SweepR97 -> SweepL73 [order 4] : after(1.923342-(kim-tim),sec)[i==1]
  SweepL73 -> latch129 [order 2] : [cellin==0 && i==0 && ctype==2]
  latch130 -> SweepL72
  SweepL79 -> SweepR105 [order 3] : after(1.5,sec)[i==0]
  SweepL79 -> SweepR105 [order 4] : after(1.5-(kim-tim),sec)[i==1]
  SweepR104 -> time145 [order 1] : [c==4]
  time145 -> SweepR104
  SweepL72 -> SweepR97 [order 4] : after(1.42-(kim-tim),sec)[i==1]
  SweepR97 -> SweepL73 [order 3] : after(1.923342,sec)[i==0]
  SweepL72 -> SweepR97 [order 3] : after(1.42,sec)[i==0]
  SweepL72 -> latch130 [order 2] : [cellin==0 && i==0 && ctype==2]
  latch129 -> SweepL73
  time131 -> SweepL73
  SweepL73 -> time131 [order 1] : [c==5]
  SweepR97 -> latch132 [order 2] : [cellin==0 && i==0 && ctype==2]
  latch132 -> SweepR97
  SweepL72 -> time127 [order 1] : [c==3]
  time127 -> SweepL72
  SweepR104 -> SweepL79 [order 4] : after(1.923342-(kim-tim),sec)[i==1]
  SweepL79 -> latch144 [order 2] : [cellin==0 && i==0 && ctype==2]
  latch141 -> SweepL80
  SweepL80 -> SweepR104 [order 4] : after(1.42-(kim-tim),sec)[i==1]
  SweepR104 -> SweepL79 [order 3] : after(1.923342,sec)[i==0]
  SweepL80 -> SweepR104 [order 3] : after(1.42,sec)[i==0]
  SweepL80 -> latch141 [order 2] : [cellin==0 && i==0 && ctype==2]
  latch144 -> SweepL79
  time143 -> SweepL79
  SweepL79 -> time143 [order 1] : [c==5]
  SweepR104 -> latch143 [order 2] : [cellin==0 && i==0 && ctype==2]
  latch143 -> SweepR104
  SweepL80 -> time142 [order 1] : [c==3]
  time142 -> SweepL80
  data: Rmotor output; Lmotor output; ang input; scolev output; ctype input; lach output; i local; time input; k local; t local; c local; tim local; kim local; cellin local; vac output; VCheck local

== matlab function AutonomousTemplate_2020a/BEST Robotics 2020 Game (Double-Click)/Vaccines/Vaccine1/MATLAB Function1 ==
  settings: updateMethod=DISCRETE
  data: drop input; level input; objPoseX output; robotPoseX input; robotPoseY input; objPoseY output; vaccine output
function [objPoseX, objPoseY, vaccine] = latchObject(drop, level, robotPoseX, robotPoseY)
persistent stateX stateY stateZ prevDrop dropped
if isempty(stateX)
    stateX=robotPoseX+0.14;
    stateY=robotPoseY;
    stateZ=0.15;
    prevDrop=0;
    dropped=0;
end

if drop && prevDrop && ~dropped
    stateX=robotPoseX;
    stateY=robotPoseY;
    stateZ=level*0.4;
    objPoseX=robotPoseX;
    objPoseY=robotPoseY;
    dropped=1;
elseif dropped
    objPoseX=stateX;
    objPoseY=stateY;

else
    objPoseX=robotPoseX-0.11;
    objPoseY=robotPoseY-0.11;
end
prevDrop=drop;
vaccine=stateZ;
